simulink model "environment_sim"  (R2019b)
settings: Solver=ode4  StartTime=0.0  StopTime=7000  FixedStep=1  RelTol=1e-3
values from neighbouring files (symbols this model uses):
  P_E =     [P_E.mat]
libraries: vrlib x2, simulink x1
settings Model: Creator=ggarrett  LastModifiedBy=ggarrett

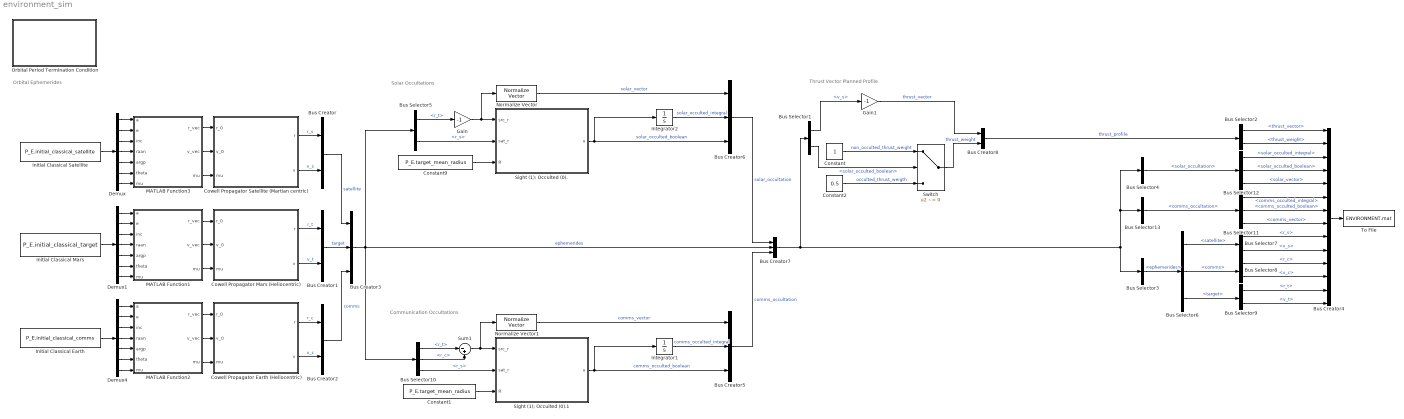
== system environment_sim ==
  note: Thrust Vector Planned Profile
  note: Solar Occultations
  note: Communication Occultations
  note: Orbital Ephemerides
  Bus Creator{,1..2,8} (4 alike) : BusCreator  Inputs=2
  Bus Creator{3,5..7} (4 alike) : BusCreator  Inputs=3
  Bus Creator4 : BusCreator  Inputs=14
  Bus Selector1 : BusSelector  OutputSignals=ephemerides.satellite.v_s,solar_occultation.solar_occulted_boolean
  Bus Selector10 : BusSelector  OutputSignals=target.r_t,comms.r_c,satellite.r_s
  Bus Selector11 : BusSelector  OutputSignals=comms_occulted_integral,comms_occulted_boolean,comms_vector
  Bus Selector12 : BusSelector  OutputSignals=solar_occulted_integral,solar_occulted_boolean,solar_vector
  Bus Selector13 : BusSelector  OutputSignals=comms_occultation
  Bus Selector2 : BusSelector  OutputSignals=thrust_vector,thrust_weight
  Bus Selector3 : BusSelector  OutputSignals=ephemerides
  Bus Selector4 : BusSelector  OutputSignals=solar_occultation
  Bus Selector5 : BusSelector  OutputSignals=target.r_t,satellite.r_s
  Bus Selector6 : BusSelector  OutputSignals=satellite,comms,target
  Bus Selector7 : BusSelector  OutputSignals=r_s,v_s
  Bus Selector8 : BusSelector  OutputSignals=r_c,v_c
  Bus Selector9 : BusSelector  OutputSignals=r_t,v_t
  Constant : Constant
  Constant1 : Constant  Value=P_E.target_mean_radius
  Constant2 : Constant  Value=0.5
  Constant9 : Constant  Value=P_E.target_mean_radius
  Cowell Propagator Earth (Heliocentric) : Subsystem
  Cowell Propagator Mars (Heliocentric) : Subsystem
  Cowell Propagator Satellite (Martian centric) : Subsystem
  Demux : Demux  Outputs=7
  Demux1 : Demux  Outputs=7
  Demux4 : Demux  Outputs=7
  Gain : Gain  Gain=-1
  Gain1 : Gain  Gain=-1
  Initial Classical Earth : Constant  Value=P_E.initial_classical_comms
  Initial Classical Mars : Constant  Value=P_E.initial_classical_target  VectorParams1D=off
  "Initial Classical Satellite " : Constant  Value=P_E.initial_classical_satellite
  Integrator1 : Integrator
  Integrator2 : Integrator
  MATLAB Function1 : MATLAB Function  TreatAsAtomicUnit=on
  MATLAB Function2 : MATLAB Function  TreatAsAtomicUnit=on
  MATLAB Function3 : MATLAB Function  TreatAsAtomicUnit=on
  Normalize Vector : vrlib/Utilities/Normalize Vector  maxzero=0
      settings: SourceProductName=Simulink
  Normalize Vector1 : vrlib/Utilities/Normalize Vector  maxzero=0
      settings: SourceProductName=Simulink
  Orbital Period Termination Condition : Subsystem
  Sight (1); Occulted (0). : MATLAB Function  TreatAsAtomicUnit=on
  Sight (1); Occulted (0).1 : MATLAB Function  TreatAsAtomicUnit=on
  Sum1 : Sum  Inputs=|-+
  Switch : Switch  Criteria=u2 ~= 0
  To File : ToFile  Filename=ENVIRONMENT.mat  MatrixName=E  SaveFormat=Timeseries
  wires:
  Initial Classical Mars/1 -> Demux1/1
  Demux/7 -> MATLAB Function3/7("mu ")
  Demux1/2 -> MATLAB Function1/2(e)
  Demux/5 -> MATLAB Function3/5(argp)
  Demux/4 -> MATLAB Function3/4(raan)
  "Initial Classical Satellite "/1 -> Demux/1
  Demux/1 -> MATLAB Function3/1(a)
  Demux/6 -> MATLAB Function3/6(theta)
  Demux1/1 -> MATLAB Function1/1(a)
  Demux1/4 -> MATLAB Function1/4(raan)
  Demux/3 -> MATLAB Function3/3(inc)
  Demux1/3 -> MATLAB Function1/3(inc)
  Demux1/5 -> MATLAB Function1/5(argp)
  Demux/2 -> MATLAB Function3/2(e)
  Demux1/6 -> MATLAB Function1/6(theta)
  Demux1/7 -> MATLAB Function1/7("mu ")
  Demux4/7 -> MATLAB Function2/7("mu ")
  Demux4/2 -> MATLAB Function2/2(e)
  Demux4/1 -> MATLAB Function2/1(a)
  Initial Classical Earth/1 -> Demux4/1
  Demux4/5 -> MATLAB Function2/5(argp)
  Demux4/3 -> MATLAB Function2/3(inc)
  Demux4/6 -> MATLAB Function2/6(theta)
  Demux4/4 -> MATLAB Function2/4(raan)
  MATLAB Function2/1(r_vec) -> Cowell Propagator Earth (Heliocentric)/1(r_0)
  MATLAB Function2/2(v_vec) -> Cowell Propagator Earth (Heliocentric)/2(v_0)
  MATLAB Function2/3(mu) -> Cowell Propagator Earth (Heliocentric)/3(mu)
  MATLAB Function1/1(r_vec) -> Cowell Propagator Mars (Heliocentric)/1(r_0)
  MATLAB Function1/2(v_vec) -> Cowell Propagator Mars (Heliocentric)/2(v_0)
  MATLAB Function1/3(mu) -> Cowell Propagator Mars (Heliocentric)/3(mu)
  MATLAB Function3/3(mu) -> Cowell Propagator Satellite (Martian centric)/3(mu)
  MATLAB Function3/2(v_vec) -> Cowell Propagator Satellite (Martian centric)/2(v_0)
  MATLAB Function3/1(r_vec) -> Cowell Propagator Satellite (Martian centric)/1(r_0)
  Constant9/1 -> Sight (1); Occulted (0)./3(R)
  Sight (1); Occulted (0)./1(u) -> Integrator2/1, Bus Creator6/3  "solar_occulted_boolean"
  Cowell Propagator Satellite (Martian centric)/1(r) -> Bus Creator/1  "r_s"
  Cowell Propagator Satellite (Martian centric)/2(v) -> Bus Creator/2  "v_s"
  Cowell Propagator Earth (Heliocentric)/1(r) -> Bus Creator2/1  "r_c"
  Cowell Propagator Earth (Heliocentric)/2(v) -> Bus Creator2/2  "v_c"
  Cowell Propagator Mars (Heliocentric)/2(v) -> Bus Creator1/2  "v_t"
  Cowell Propagator Mars (Heliocentric)/1(r) -> Bus Creator1/1  "r_t"
  Bus Creator/1 -> Bus Creator3/1  "satellite"
  Bus Creator1/1 -> Bus Creator3/2  "target"
  Bus Creator2/1 -> Bus Creator3/3  "comms"
  Bus Creator3/1 -> Bus Creator7/2, Bus Selector5/1, Bus Selector10/1  "ephemerides"
  Bus Selector5/2 -> Sight (1); Occulted (0)./2(sat_r)  "<r_s>"
  Bus Selector5/1 -> Gain/1  "<r_t>"
  Gain/1 -> Normalize Vector/1, Sight (1); Occulted (0)./1(src_r)
  Sight (1); Occulted (0).1/1(u) -> Bus Creator5/3, Integrator1/1  "comms_occulted_boolean"
  Bus Selector10/1 -> Sum1/1  "<r_t>"
  Sum1/1 -> Normalize Vector1/1, Sight (1); Occulted (0).1/1(src_r)
  Bus Selector10/3 -> Sight (1); Occulted (0).1/2(sat_r)  "<r_s>"
  Constant1/1 -> Sight (1); Occulted (0).1/3(R)
  Bus Selector10/2 -> Sum1/2  "<r_c>"
  Normalize Vector/1 -> Bus Creator6/1  "solar_vector"
  Normalize Vector1/1 -> Bus Creator5/1  "comms_vector"
  Bus Selector1/1 -> Gain1/1  "<v_s>"
  Bus Creator4/1 -> To File/1
  Gain1/1 -> Bus Creator8/1  "thrust_vector"
  Integrator1/1 -> Bus Creator5/2  "comms_occulted_integral"
  Integrator2/1 -> Bus Creator6/2  "solar_occulted_integral"
  Bus Creator5/1 -> Bus Creator7/3  "comms_occultation"
  Bus Creator7/1 -> Bus Selector4/1, Bus Selector13/1, Bus Selector3/1, Bus Selector1/1
  Bus Creator6/1 -> Bus Creator7/1  "solar_occultation"
  Constant/1 -> Switch/1  "non_occulted_thrust_weight"
  Constant2/1 -> Switch/3  "occulted_thrust_weigth"
  Switch/1 -> Bus Creator8/2  "thrust_weight"
  Bus Selector6/2 -> Bus Selector8/1  "<comms>"
  Bus Selector7/2 -> Bus Creator4/10  "<v_s>"
  Bus Selector9/1 -> Bus Creator4/13  "<r_t>"
  Bus Selector8/2 -> Bus Creator4/12  "<v_c>"
  Bus Selector6/3 -> Bus Selector9/1  "<target>"
  Bus Selector8/1 -> Bus Creator4/11  "<r_c>"
  Bus Selector6/1 -> Bus Selector7/1  "<satellite>"
  Bus Selector9/2 -> Bus Creator4/14  "<v_t>"
  Bus Selector7/1 -> Bus Creator4/9  "<r_s>"
  Bus Selector2/1 -> Bus Creator4/1  "<thrust_vector>"
  Bus Creator8/1 -> Bus Selector2/1  "thrust_profile"
  Bus Selector2/2 -> Bus Creator4/2  "<thrust_weight>"
  Bus Selector4/1 -> Bus Selector12/1  "<solar_occultation>"
  Bus Selector12/1 -> Bus Creator4/3  "<solar_occulted_integral>"
  Bus Selector12/2 -> Bus Creator4/4  "<solar_occulted_boolean>"
  Bus Selector11/2 -> Bus Creator4/7  "<comms_occulted_boolean>"
  Bus Selector13/1 -> Bus Selector11/1  "<comms_occultation>"
  Bus Selector11/1 -> Bus Creator4/6  "<comms_occulted_integral>"
  Bus Selector3/1 -> Bus Selector6/1  "<ephemerides>"
  Bus Selector1/2 -> Switch/2  "<solar_occulted_boolean>"
  Bus Selector12/3 -> Bus Creator4/5  "<solar_vector>"
  Bus Selector11/3 -> Bus Creator4/8  "<comms_vector>"

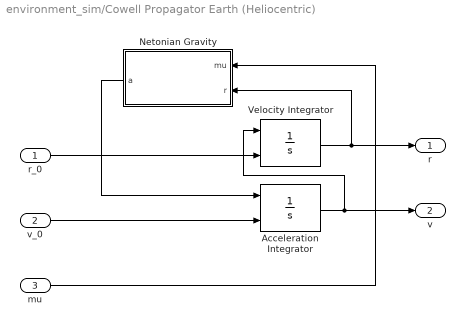
== system environment_sim/Cowell Propagator Earth (Heliocentric) ==
  r_0 : Inport
  v_0 : Inport  Port=2
  mu : Inport  Port=3
  Acceleration Integrator : Integrator  InitialConditionSource=external
  Netonian Gravity : MATLAB Function  TreatAsAtomicUnit=on
  Velocity Integrator : Integrator  InitialConditionSource=external
  r : Outport
  v : Outport  Port=2
  wires:
  Acceleration Integrator/1 -> v/1, Velocity Integrator/1
  v_0/1 -> Acceleration Integrator/2
  Velocity Integrator/1 -> r/1, Netonian Gravity/2(r)
  Netonian Gravity/1(a) -> Acceleration Integrator/1
  r_0/1 -> Velocity Integrator/2
  mu/1 -> Netonian Gravity/1(mu)

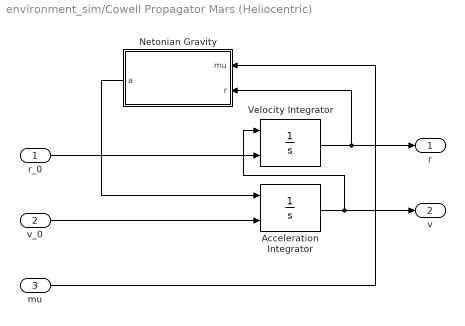
== system environment_sim/Cowell Propagator Mars (Heliocentric) ==
  r_0 : Inport
  v_0 : Inport  Port=2
  mu : Inport  Port=3
  Acceleration Integrator : Integrator  InitialConditionSource=external
  Netonian Gravity : MATLAB Function  TreatAsAtomicUnit=on
  Velocity Integrator : Integrator  InitialConditionSource=external
  r : Outport
  v : Outport  Port=2
  wires:
  Acceleration Integrator/1 -> v/1, Velocity Integrator/1
  v_0/1 -> Acceleration Integrator/2
  Velocity Integrator/1 -> r/1, Netonian Gravity/2(r)
  Netonian Gravity/1(a) -> Acceleration Integrator/1
  r_0/1 -> Velocity Integrator/2
  mu/1 -> Netonian Gravity/1(mu)

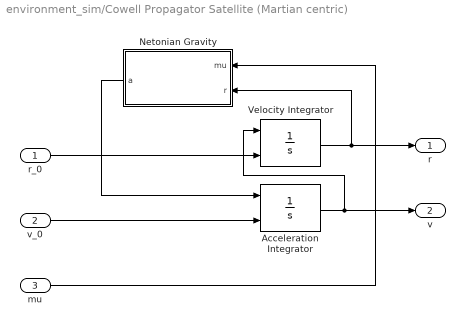
== system environment_sim/Cowell Propagator Satellite (Martian centric) ==
  r_0 : Inport
  v_0 : Inport  Port=2
  mu : Inport  Port=3
  Acceleration Integrator : Integrator  InitialConditionSource=external
  Netonian Gravity : MATLAB Function  TreatAsAtomicUnit=on
  Velocity Integrator : Integrator  InitialConditionSource=external
  r : Outport
  v : Outport  Port=2
  wires:
  Acceleration Integrator/1 -> v/1, Velocity Integrator/1
  v_0/1 -> Acceleration Integrator/2
  Velocity Integrator/1 -> r/1, Netonian Gravity/2(r)
  Netonian Gravity/1(a) -> Acceleration Integrator/1
  r_0/1 -> Velocity Integrator/2
  mu/1 -> Netonian Gravity/1(mu)

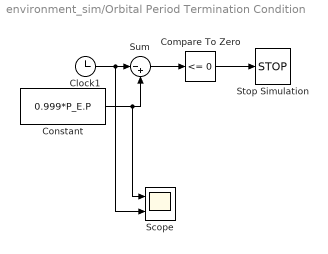
== system environment_sim/Orbital Period Termination Condition ==
  Clock1 : Clock
  Compare To Zero : simulink/Logic and Bit Operations/Compare To Zero  relop=<=  OutDataTypeStr=boolean
  Constant : Constant  Value=0.999*P_E.P
  Scope : Scope  NumInputPorts=2
  Stop Simulation : Stop
  Sum : Sum  Inputs=|-+
  wires:
  Constant/1 -> Scope/1, Sum/2
  Clock1/1 -> Scope/2, Sum/1
  Sum/1 -> Compare To Zero/1
  Compare To Zero/1 -> Stop Simulation/1

== matlab function environment_sim/MATLAB Function3 ==
  data: a input; r_vec output; e input; inc input; raan input; argp input; theta input; mu input; v_vec output; mu output
function [r_vec,v_vec, mu] = coe2rv(a, e, inc, raan, argp, theta, mu)
    cos_raan = cos(raan);
    sin_raan = sin(raan);
    cos_argp = cos(argp);
    sin_argp = sin(argp);
    cos_inc = cos(inc);
    sin_inc = sin(inc);
    r = a * (1 - e ^ 2) / (1.0 + e * cos(theta));

    l1 = (+cos_raan * cos_argp - sin_raan * sin_argp * cos_inc);
    l2 = (-cos_raan * sin_argp - sin_raan * cos_argp * cos_inc);
    m1 = (+sin_raan * cos_argp + cos_raan * sin_argp * cos_inc);
    m2 = (-sin_raan * sin_argp + cos_raan * cos_argp * cos_inc);
    n1 = sin_argp * sin_inc;
    n2 = cos_argp * sin_inc;

    aux = [r * cos(theta); r * sin(theta)];
    transformation = [l1, l2;...
                      m1, m2;...
                      n1, n2];

    % Position
    xyz = transformation * aux;
    x = xyz(1);
    y = xyz(2);
    z = xyz(3);

    % Velocity
    H = sqrt(mu * a * (1 - e ^ 2));
    v_x = mu / H * (-l1 * sin(theta) + l2 * (e + cos(theta)));
    v_y = mu / H * (-m1 * sin(theta) + m2 * (e + cos(theta)));
    v_z = mu / H * (-n1 * sin(theta) + n2 * (e + cos(theta)));
    r_vec = [x; y; z];
    v_vec = [v_x; v_y; v_z];
end

== matlab function environment_sim/Cowell Propagator Earth (Heliocentric)/Netonian Gravity ==
  data: mu input; r input; a output
function a = newtonGrav(mu, r)

a = -(mu / norm(r)^3) * r;

== matlab function environment_sim/MATLAB Function2 ==
  data: a input; r_vec output; e input; inc input; raan input; argp input; theta input; mu input; v_vec output; mu output
function [r_vec,v_vec, mu] = coe2rv(a, e, inc, raan, argp, theta, mu)
    cos_raan = cos(raan);
    sin_raan = sin(raan);
    cos_argp = cos(argp);
    sin_argp = sin(argp);
    cos_inc = cos(inc);
    sin_inc = sin(inc);
    r = a * (1 - e ^ 2) / (1.0 + e * cos(theta));

    l1 = (+cos_raan * cos_argp - sin_raan * sin_argp * cos_inc);
    l2 = (-cos_raan * sin_argp - sin_raan * cos_argp * cos_inc);
    m1 = (+sin_raan * cos_argp + cos_raan * sin_argp * cos_inc);
    m2 = (-sin_raan * sin_argp + cos_raan * cos_argp * cos_inc);
    n1 = sin_argp * sin_inc;
    n2 = cos_argp * sin_inc;

    aux = [r * cos(theta); r * sin(theta)];
    transformation = [l1, l2;...
                      m1, m2;...
                      n1, n2];

    % Position
    xyz = transformation * aux;
    x = xyz(1);
    y = xyz(2);
    z = xyz(3);

    % Velocity
    H = sqrt(mu * a * (1 - e ^ 2));
    v_x = mu / H * (-l1 * sin(theta) + l2 * (e + cos(theta)));
    v_y = mu / H * (-m1 * sin(theta) + m2 * (e + cos(theta)));
    v_z = mu / H * (-n1 * sin(theta) + n2 * (e + cos(theta)));
    r_vec = [x; y; z];
    v_vec = [v_x; v_y; v_z];
end

== matlab function environment_sim/MATLAB Function1 ==
  data: a input; r_vec output; e input; inc input; raan input; argp input; theta input; mu input; v_vec output; mu output
function [r_vec,v_vec, mu] = coe2rv(a, e, inc, raan, argp, theta, mu)
    cos_raan = cos(raan);
    sin_raan = sin(raan);
    cos_argp = cos(argp);
    sin_argp = sin(argp);
    cos_inc = cos(inc);
    sin_inc = sin(inc);
    r = a * (1 - e ^ 2) / (1.0 + e * cos(theta));

    l1 = (+cos_raan * cos_argp - sin_raan * sin_argp * cos_inc);
    l2 = (-cos_raan * sin_argp - sin_raan * cos_argp * cos_inc);
    m1 = (+sin_raan * cos_argp + cos_raan * sin_argp * cos_inc);
    m2 = (-sin_raan * sin_argp + cos_raan * cos_argp * cos_inc);
    n1 = sin_argp * sin_inc;
    n2 = cos_argp * sin_inc;

    aux = [r * cos(theta); r * sin(theta)];
    transformation = [l1, l2;...
                      m1, m2;...
                      n1, n2];

    % Position
    xyz = transformation * aux;
    x = xyz(1);
    y = xyz(2);
    z = xyz(3);

    % Velocity
    H = sqrt(mu * a * (1 - e ^ 2));
    v_x = mu / H * (-l1 * sin(theta) + l2 * (e + cos(theta)));
    v_y = mu / H * (-m1 * sin(theta) + m2 * (e + cos(theta)));
    v_z = mu / H * (-n1 * sin(theta) + n2 * (e + cos(theta)));
    r_vec = [x; y; z];
    v_vec = [v_x; v_y; v_z];
end

== matlab function environment_sim/Cowell Propagator Mars (Heliocentric)/Netonian Gravity ==
  data: mu input; r input; a output
function a = newtonGrav(mu, r)

a = -(mu / norm(r)^3) * r;

== matlab function environment_sim/Cowell Propagator Satellite (Martian centric)/Netonian Gravity ==
  data: mu input; r input; a output
function a = newtonGrav(mu, r)

a = -(mu / norm(r)^3) * r;

== matlab function environment_sim/Sight (1); Occulted (0). ==
  data: src_r input; u output; sat_r input; R input
function u = sight_function(src_r, sat_r, R)
% Parameters
% ----------
% src_v : double, shape=(1,3)
%   source vector which is being checked for occultation by
%   planet of radius rad_p. Origin of vector is center of planet.
% sat_r : double, shape=(1,3)
%   inertial vector of satellite orbiting planet.
% R : double
%   radius of the planet being orbited.
spacecraft_h = norm(sat_r) - R; % Calculate spacecraft h.
src_v = src_r/norm(src_r);      % Source unit vector.
sat_v = sat_r/norm(sat_r);      % Satellite unit vector.
cos_phi = dot(src_v, sat_v);
a_sin_phi = (R + spacecraft_h) * sin(acos(cos_phi));
if (cos_phi < 0) && (a_sin_phi <R)
    u=0;   % Occulted (signal is blocked).
else
    u=1;   % Not occulted (allows signal to pass).
end

== matlab function environment_sim/Sight (1); Occulted (0).1 ==
  data: src_r input; u output; sat_r input; R input
function u = sight_function(src_r, sat_r, R)
% Parameters
% ----------
% src_v : double, shape=(1,3)
%   source vector which is being checked for occultation by
%   planet of radius rad_p. Origin of vector is center of planet.
% sat_r : double, shape=(1,3)
%   inertial vector of satellite orbiting planet.
% R : double
%   radius of the planet being orbited.
spacecraft_h = norm(sat_r) - R; % Calculate spacecraft h.
src_v = src_r/norm(src_r);      % Source unit vector.
sat_v = sat_r/norm(sat_r);      % Satellite unit vector.
cos_phi = dot(src_v, sat_v);
a_sin_phi = (R + spacecraft_h) * sin(acos(cos_phi));
if (cos_phi < 0) && (a_sin_phi <R)
    u=0;   % Occulted (signal is blocked).
else
    u=1;   % Not occulted (allows signal to pass).
end
